simulink model "d4"  (R2014b)
settings: Solver=ode45  StartTime=0.0  StopTime=10  RelTol=1e-3
settings Model: Creator=Ashish  LastModifiedBy=Ashish

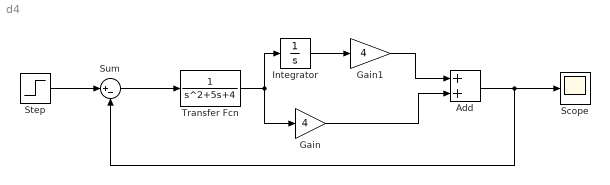
== system d4 ==
  Add : Sum
  Gain : Gain  Gain=4
  Gain1 : Gain  Gain=4
  Integrator : Integrator
  Scope : Scope
      settings: TimeRange=100
  Step : Step  Time=0  SampleTime=0
  Sum : Sum  Inputs=|+-
  Transfer Fcn : TransferFcn  Denominator=[1 5 4]
  wires:
  Step/1 -> Sum/1
  Sum/1 -> Transfer Fcn/1
  Transfer Fcn/1 -> Integrator/1, Gain/1
  Gain/1 -> Add/2
  Add/1 -> Sum/2, Scope/1
  Integrator/1 -> Gain1/1
  Gain1/1 -> Add/1
